simulink model "pendulum_system"  (R2025b)
settings: Solver=VariableStepAuto  StartTime=0.0  StopTime=3  RelTol=1e-3
undefined symbols (not defined in the file): g0, g1, h
libraries: fuzblock x1
settings Model: Creator=brianli  LastModifiedBy=brianli

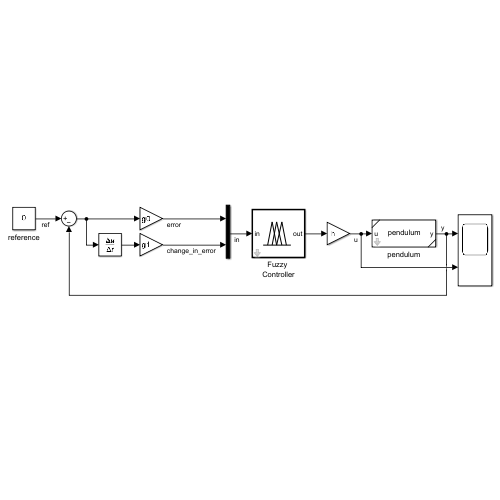
[thumbnail: Simulink's stored preview of the top-level diagram]
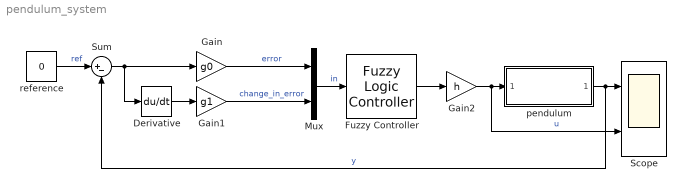
== system pendulum_system ==
  Derivative : Derivative  CoefficientInTFapproximation=1e3
  Fuzzy Controller : fuzblock/Fuzzy Logic  Controller  FIS=pendulum_ctrl_triangular  OutputSampleNumber=101  DataType=double  UseLookupTable=off  NumBreakpoints=10  FuzzifiedInputs=off  RuleFiringStrengths=off  RuleOutputs=off  AggregatedOutputs=off  SimulateUsing=Interpreted execution  OutOfRangeInputValueMessage=warning  NoRuleFiredMessage=warning  EmptyOutputFuzzySetMessage=warning
  Gain : Gain  Gain=g0
  Gain1 : Gain  Gain=g1
  Gain2 : Gain  Gain=h
  Mux : Mux  Inputs=2
  Scope : Scope  NumInputPorts=2
      settings: ActiveDisplayYMinimum=-0.0053029096496502205  ActiveDisplayYMaximum=0.11240537316713407
  Sum : Sum  Inputs=|+-
  pendulum : Subsystem  ReferencedSubsystem=pendulum  y0=0.1  dy0=0  u0=0
  reference : Constant  Value=0
  wires:
  reference/1 -> Sum/1  "ref"
  Mux/1 -> Fuzzy Controller/1  "in"
  Sum/1 -> Gain/1, Derivative/1
  pendulum/1 -> Sum/2, Scope/1  "y"
  Fuzzy Controller/1 -> Gain2/1
  Gain1/1 -> Mux/2  "change_in_error"
  Gain/1 -> Mux/1  "error"
  Derivative/1 -> Gain1/1
  Gain2/1 -> Scope/2, pendulum/1  "u"
